simulink model "Integrator_Block_Implemntation"  (R2024a)
settings: Solver=FixedStepAuto  StartTime=0.0  StopTime=10.0  RelTol=1e-3
undefined symbols (not defined in the file or in its folder): DiscIntNeverNeededParam
libraries: simulink x1
settings Model: Creator=VICTUS  LastModifiedBy=VICTUS

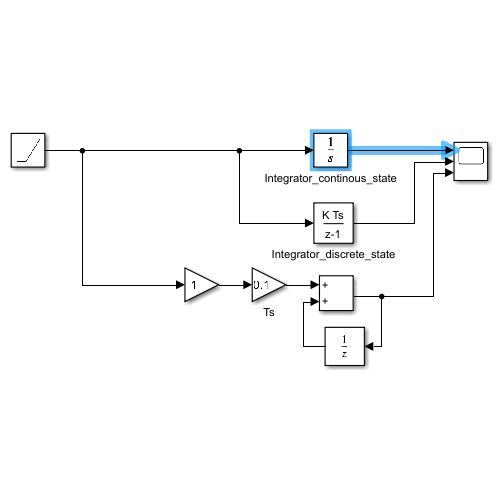
[thumbnail: Simulink's stored preview of the top-level diagram]
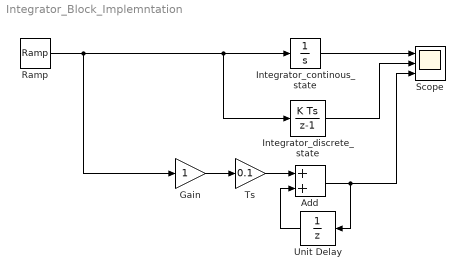
== system Integrator_Block_Implemntation ==
  Add : Sum
  Gain : Gain
  Integrator_continous_state : Integrator
  Integrator_discrete_state : DiscreteIntegrator  SampleTime=0.1  ICPrevOutput=DiscIntNeverNeededParam  ICPrevScaledInput=DiscIntNeverNeededParam
  Ramp : simulink/Sources/Ramp  slope=1  start=0  InitialOutput=0
  Scope : Scope  NumInputPorts=3
  Ts : Gain  Gain=0.1
  Unit Delay : UnitDelay  SampleTime=-1  HasFrameUpgradeWarning=on
  wires:
  Integrator_continous_state/1 -> Scope/1
  Integrator_discrete_state/1 -> Scope/2
  Add/1 -> Scope/3, Unit Delay/1
  Unit Delay/1 -> Add/2
  Ts/1 -> Add/1
  Gain/1 -> Ts/1
  Ramp/1 -> Gain/1, Integrator_continous_state/1, Integrator_discrete_state/1
